simulink model "Turbine"  (R2024a)
settings: Solver=ode1  StartTime=0.0  StopTime=50  FixedStep=0.0001  RelTol=1e-3
InitFcn:
  | ng       = 97;
settings Model: Creator=user  LastModifiedBy=anif4
settings RTWCC: GPUComputeCapability=3.5

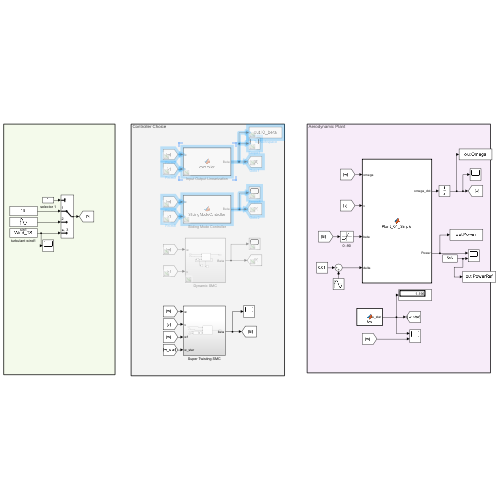
[thumbnail: Simulink's stored preview of the top-level diagram]
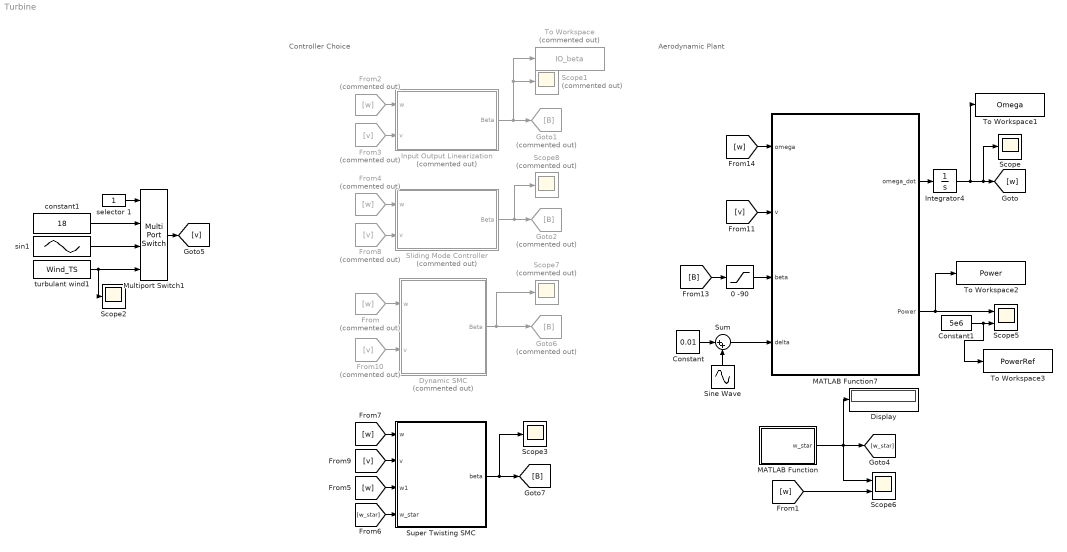
== system Turbine ==
  note: Controller Choice
  note: Aerodynamic Plant
  0 -90 : Saturate  UpperLimit=90  LowerLimit=0
  Constant : Constant  Value=0.01
  Constant1 : Constant  Value=5e6
  Display : Display
  Dynamic SMC : Subsystem  Commented=on
  From : From  Commented=on  GotoTag=w
  From10 : From  Commented=on  GotoTag=v
  From2 : From  Commented=on  GotoTag=w
  From3 : From  Commented=on  GotoTag=v
  From4 : From  Commented=on  GotoTag=w
  From8 : From  Commented=on  GotoTag=v
  Goto1 : Goto  Commented=on  GotoTag=B
  Goto2 : Goto  Commented=on  GotoTag=B
  Goto6 : Goto  Commented=on  GotoTag=B
  Input Output Linearization : MATLAB Function  Commented=on  TreatAsAtomicUnit=on
  Integrator4 : Integrator  InitialCondition=2
  MATLAB Function : MATLAB Function  TreatAsAtomicUnit=on
  MATLAB Function7 : MATLAB Function  TreatAsAtomicUnit=on
  Multiport Switch1 : MultiPortSwitch  SaturateOnIntegerOverflow=off  InputSameDT=off
  Scope : Scope
  Scope1 : Scope  Commented=on
  Scope2 : Scope
  Scope3 : Scope
  Scope5 : Scope  NumInputPorts=2
  Scope6 : Scope  NumInputPorts=2
  Scope7 : Scope  Commented=on
  Scope8 : Scope  Commented=on
  Sine Wave : Sin  Amplitude=0.2  Frequency=0.5  SampleTime=0
  Sliding Mode Controller : MATLAB Function  Commented=on  TreatAsAtomicUnit=on
  Sum : Sum  Inputs=|++
  Super Twisting SMC : Subsystem
  To Workspace : ToWorkspace  Commented=on  VariableName=IO_beta  SampleTime=-1
  To Workspace1 : ToWorkspace  VariableName=Omega  SampleTime=-1
  To Workspace2 : ToWorkspace  VariableName=Power  SampleTime=-1
  To Workspace3 : ToWorkspace  VariableName=PowerRef  SampleTime=-1
  constant1 : Constant  Value=18
  selector 1 : Constant
  sin1 : Sin  Bias=20  Frequency=0.5  SampleTime=0
  turbulant wind1 : FromWorkspace  VariableName=Wind_TS
  wires:
  selector 1/1 -> Multiport Switch1/1
  constant1/1 -> Multiport Switch1/2
  sin1/1 -> Multiport Switch1/3
  Multiport Switch1/1 -> [v]
  MATLAB Function7/2(Power) -> To Workspace2/1, Scope5/1
  turbulant wind1/1 -> Scope2/1, Multiport Switch1/4
  MATLAB Function7/1(omega_dot) -> Integrator4/1
  Constant1/1 -> To Workspace3/1, Scope5/2
  Integrator4/1 -> To Workspace1/1, Scope/1, [w]
  Sum/1 -> MATLAB Function7/4(delta)
  Constant/1 -> Sum/1
  Sine Wave/1 -> Sum/2
  MATLAB Function/1(w_star) -> Display/1, Scope6/1, [w_star]
  [w] -> Scope6/2
  0 -90/1 -> MATLAB Function7/3(beta)
  [v] -> MATLAB Function7/2(v)
  [B] -> 0 -90/1
  [w] -> MATLAB Function7/1(omega)
  [w] -> Super Twisting SMC/1(w)
  [v] -> Super Twisting SMC/2(v)
  [w] -> Super Twisting SMC/3(w1)
  [w_star] -> Super Twisting SMC/4(w_star)
  Super Twisting SMC/1(beta) -> Scope3/1, [B]
  From/1 -> Dynamic SMC/1(w)
  From10/1 -> Dynamic SMC/2(v)
  Dynamic SMC/1(Beta) -> Goto6/1, Scope7/1
  Input Output Linearization/1(Beta) -> Goto1/1, To Workspace/1, Scope1/1
  From2/1 -> Input Output Linearization/1(w)
  From3/1 -> Input Output Linearization/2(v)
  From8/1 -> Sliding Mode Controller/2(v)
  From4/1 -> Sliding Mode Controller/1(w)
  Sliding Mode Controller/1(Beta) -> Goto2/1, Scope8/1

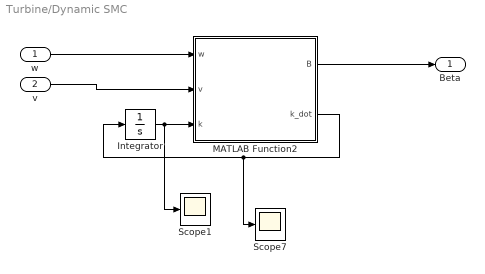
== system Turbine/Dynamic SMC ==
  w : Inport
  v : Inport  Port=2
  Integrator : Integrator
  MATLAB Function2 : MATLAB Function  TreatAsAtomicUnit=on
  Scope1 : Scope
  Scope7 : Scope
  Beta : Outport
  wires:
  Integrator/1 -> MATLAB Function2/3(k), Scope1/1
  MATLAB Function2/2(k_dot) -> Scope7/1, Integrator/1
  w/1 -> MATLAB Function2/1(w)
  MATLAB Function2/1(B) -> Beta/1
  v/1 -> MATLAB Function2/2(v)

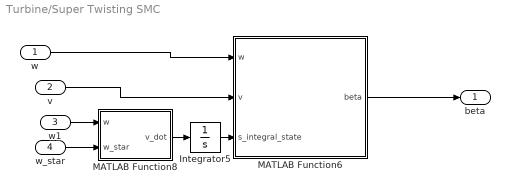
== system Turbine/Super Twisting SMC ==
  w : Inport
  v : Inport  Port=2
  w1 : Inport  Port=3
  w_star : Inport  Port=4
  Integrator5 : Integrator
  MATLAB Function6 : MATLAB Function  TreatAsAtomicUnit=on
  MATLAB Function8 : MATLAB Function  TreatAsAtomicUnit=on
  beta : Outport
  wires:
  MATLAB Function8/1(v_dot) -> Integrator5/1
  Integrator5/1 -> MATLAB Function6/3(s_integral_state)
  w/1 -> MATLAB Function6/1(w)
  w_star/1 -> MATLAB Function8/2(w_star)
  w1/1 -> MATLAB Function8/1(w)
  MATLAB Function6/1(beta) -> beta/1
  v/1 -> MATLAB Function6/2(v)

== matlab function Turbine/Input Output Linearization ==
  data: w input; Beta output; v input
function Beta  = controller(w,v)

% Parameters
ng       = 97;
taugStar = 43093;      % N.m (generator rated torque)
R        = 63;         % m
rho      = 1.22;       % kg/m^3
J        = 38759228;   % kg.m^2

% Tip-speed ratio
lambda = (w * R) / v;  
k=45;
% Coefficients
c0 = 0.5;  c1 = 73.5; c2 = 0.4; c3 = 5;
c4 = 13.125; c5 = 0.08; c6 = 0.035;
u=20;
% Aerodynamic Cp approximation (depends on lambda and beta)
lambda1_inv = 1/(lambda + c5*u) - c6/(u^3 + 1);
a = -(c0*c2) * exp(-c4*lambda1_inv);
b =  (c0*(c1*lambda1_inv - c3)) * exp(-c4*lambda1_inv);
Cp = a*u + b;      % Cp in affine-form w.r.t. beta
Cp = min(max(Cp, 0), 0.5);

n_g=97; %Gearbox ratio
t_g=4.309355*10^4;  %Rated generator torque
P_star=5*10^6; % Rated electrical power

w_star=P_star/(n_g*t_g);
e = w - w_star;
e_dot=-k*e;
F = (1/J) * ( ((0.5 * rho * pi * R^3 * v^2)/lambda)*b - ng*taugStar );
G = (1/J) * ( ((0.5 * rho * pi * R^3 * v^2)/lambda)*a );

Beta= (-F+e_dot)/G;

end

== matlab function Turbine/Dynamic SMC/MATLAB Function2 ==
  data: w input; B output; v input; k_dot output; k input
function [B,k_dot]  = DynamicGain_SlidingModeController(w,v,k)

% Parameters
ng       = 97;
taugStar = 43093;      % N.m (generator rated torque)
R        = 63;         % m
rho      = 1.22;       % kg/m^3
J        = 38759228;   % kg.m^2
E= 0.0003;

% Tip-speed ratio
lambda = (w * R) / v;  

% Coefficients
c0 = 0.5;  c1 = 73.5; c2 = 0.4; c3 = 5;
c4 = 13.125; c5 = 0.08; c6 = 0.035;
u=20;
% Aerodynamic Cp approximation (depends on lambda and beta)
lambda1_inv = 1/(lambda + c5*u) - c6/(u^3 + 1);
a = -(c0*c2) * exp(-c4*lambda1_inv);
b =  (c0*(c1*lambda1_inv - c3)) * exp(-c4*lambda1_inv);
Cp = a*u + b;      % Cp in affine-form w.r.t. beta
Cp = min(max(Cp, 0), 0.5);

n_g=97; %Gearbox ratio
t_g=4.309355*10^4;  %Rated generator torque
P_star=5*10^6; % Rated electrical power

w_star=P_star/(n_g*t_g);
s = w - w_star;
k_dot=0.5* sign(abs(s)-E);

%e_dot=-k*e;
F = (1/J) * ( ((0.5 * rho * pi * R^3 * v^2)/lambda)*b - ng*taugStar );
G = (1/J) * ( ((0.5 * rho * pi * R^3 * v^2)/lambda)*a );

B= -(F/G)-(k*sign(s))/G;

end

== matlab function Turbine/MATLAB Function7 ==
  data: omega input; omega_dot output; v input; beta input; Power output; delta input
function [omega_dot, Power] = Plant_Q1_Simple(omega, v, beta, delta)

% Parameters
ng       = 97;
taugStar = 43093;      % N.m (generator rated torque)
R        = 63;         % m
rho      = 1.22;       % kg/m^3
J        = 38759228;   % kg.m^2

% Tip-speed ratio
lambda = (omega * R) / v;  

% Coefficients
c0 = 0.5;  c1 = 73.5; c2 = 0.4; c3 = 5;
c4 = 13.125; c5 = 0.08; c6 = 0.035;

u = beta; 

% Aerodynamic Cp approximation (depends on lambda and beta)
lambda1_inv = 1/(lambda + c5*u) - c6/(u^3 + 1);
a = -(c0*c2) * exp(-c4*lambda1_inv);
b =  (c0*(c1*lambda1_inv - c3)) * exp(-c4*lambda1_inv);
Cp = a*u + b;      % Cp in affine-form w.r.t. beta
%Cp = min(max(Cp, 0), 0.5);


% K = (0.5 * rho * pi * R^2 * v^3);  % Wind power factor


Power = taugStar * ng * omega ;   % Aerodynamic power


% ---- F + G*u form ----
F = (1/J) * ( ((0.5 * rho * pi * R^3 * v^2)/omega)*b - ng*taugStar );
G = (1/J) * ( ((0.5 * rho * pi * R^3 * v^2)/omega)*a );

omega_dot = F + G*u + delta;

end

== matlab function Turbine/Sliding Mode Controller ==
  data: w input; Beta output; v input
function Beta  = SlidingModeController(w,v)

% Parameters
ng       = 97;
taugStar = 43093;      % N.m (generator rated torque)
R        = 63;         % m
rho      = 1.22;       % kg/m^3
J        = 38759228;   % kg.m^2

% Tip-speed ratio
lambda = (w * R) / v;  
k=10;
% Coefficients
c0 = 0.5;  c1 = 73.5; c2 = 0.4; c3 = 5;
c4 = 13.125; c5 = 0.08; c6 = 0.035;
u=20;
% Aerodynamic Cp approximation (depends on lambda and beta)
lambda1_inv = 1/(lambda + c5*u) - c6/(u^3 + 1);
a = -(c0*c2) * exp(-c4*lambda1_inv);
b =  (c0*(c1*lambda1_inv - c3)) * exp(-c4*lambda1_inv);
Cp = a*u + b;      % Cp in affine-form w.r.t. beta
Cp = min(max(Cp, 0), 0.5);

n_g=97; %Gearbox ratio
t_g=4.309355*10^4;  %Rated generator torque
P_star=5*10^6; % Rated electrical power

w_star=P_star/(n_g*t_g);
s = w - w_star;
%e_dot=-k*e;
F = (1/J) * ( ((0.5 * rho * pi * R^3 * v^2)/lambda)*b - ng*taugStar );
G = (1/J) * ( ((0.5 * rho * pi * R^3 * v^2)/lambda)*a );

Beta= -(F/G)-(k*sign(s))/G;

end

== matlab function Turbine/MATLAB Function ==
  data: w_star output
function w_star = fcn()
ng       = 97;
taugStar = 43093;      % N.m (generator rated torque)
R        = 63;         % m
rho      = 1.22;       % kg/m^3
J        = 38759228;

n_g=97; %Gearbox ratio
t_g=4.309355*10^4;  %Rated generator torque
P_star=5*10^6; % Rated electrical power

w_star=P_star/(n_g*t_g);

== matlab function Turbine/Super Twisting SMC/MATLAB Function6 ==
  data: w input; beta output; v input; s_integral_state input
function beta  = SuperTwisting_Controller(w, v, s_integral_state)
% Parameters (matching your existing plant)
ng       = 97;
taugStar = 43093;      
R        = 63;         
rho      = 1.22;       
J        = 38759228;   
P_star   = 5e6;

% Calculate rated speed and sliding surface
w_star = P_star / (ng * taugStar);
s = w - w_star;

% --- Gains Selection ---
% Tune k1 and k2 based on the bound of your perturbation delta(t)
k1 = 0.58; 
k2 = 0.02;

% --- Plant Dynamics (F and G) ---
lambda = (w * R) / v;
c0 = 0.5; c1 = 73.5; c2 = 0.4; c3 = 5;
c4 = 13.125; c5 = 0.08; c6 = 0.035;

% For linearization, we use a nominal pitch (e.g., u = 20)
u_nom = 20; 
lambda1_inv = 1/(lambda + c5*u_nom) - c6/(u_nom^3 + 1);
a = -(c0*c2) * exp(-c4*lambda1_inv);
b = (c0*(c1*lambda1_inv - c3)) * exp(-c4*lambda1_inv);

F = (1/J) * ( ((0.5 * rho * pi * R^3 * v^2)/lambda)*b - ng*taugStar );
G = (1/J) * ( ((0.5 * rho * pi * R^3 * v^2)/lambda)*a );

% --- Super-Twisting Law ---
% u_sta = -k1 * |s|^0.5 * sign(s) + v_dot_integral
u_sta = -k1 * sqrt(abs(s)) * sign(s) + s_integral_state;

beta = (u_sta - F) / G;
end

== matlab function Turbine/Super Twisting SMC/MATLAB Function8 ==
  data: w input; v_dot output; w_star input
function v_dot = fcn(w, w_star)
k2 = 0.02;
s = w - w_star;

v_dot = -k2*sign(s);


end
